simulink model "duality"  (Simulink 7.3)
settings: Solver=FixedStepDiscrete  StartTime=0.0  StopTime=10.0  FixedStep=0.02  RelTol=1e-3
libraries: voderiv x8
settings Model: Creator=Dominik  LastModifiedBy=dominik

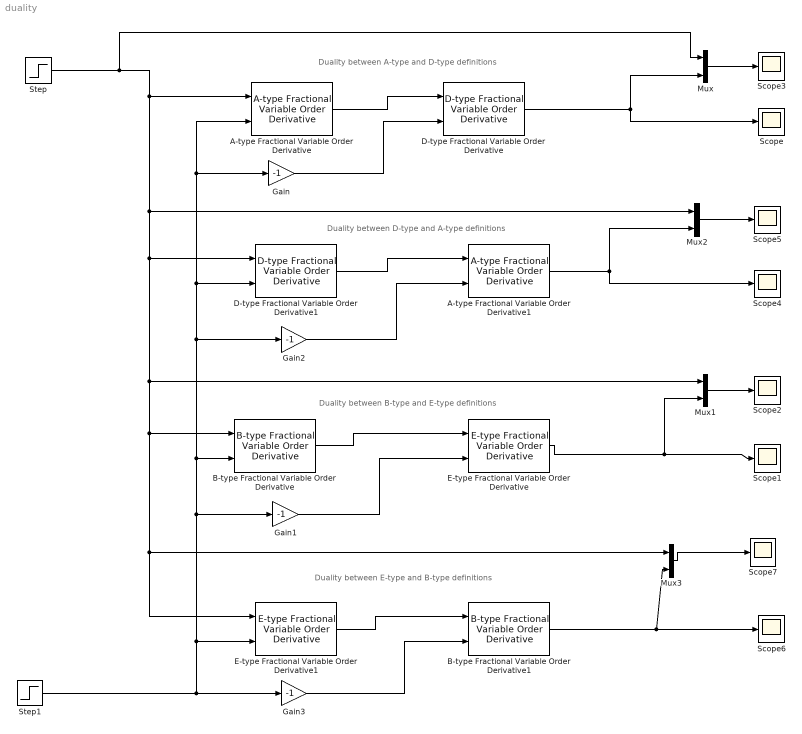
== system duality ==
  note: Duality between A-type and D-type definitions
  note: Duality between D-type and A-type definitions
  note: Duality between B-type and E-type definitions
  note: Duality between E-type and B-type definitions
  A-type Fractional Variable Order Derivative : voderiv/A-type Fractional Variable Order Derivative  N=1  Nbuf=500  Ts=0.02
  A-type Fractional Variable Order Derivative1 : voderiv/A-type Fractional Variable Order Derivative  N=1  Nbuf=500  Ts=0.02
  B-type Fractional Variable Order Derivative : voderiv/B-type Fractional Variable Order Derivative  N=1  Nbuf=500  Ts=0.02
  B-type Fractional Variable Order Derivative1 : voderiv/B-type Fractional Variable Order Derivative  N=1  Nbuf=500  Ts=0.02
  D-type Fractional Variable Order Derivative : voderiv/D-type Fractional Variable Order Derivative  N=1  Nbuf=500  Ts=0.02
  D-type Fractional Variable Order Derivative1 : voderiv/D-type Fractional Variable Order Derivative  N=1  Nbuf=500  Ts=0.02
  E-type Fractional Variable Order Derivative : voderiv/E-type Fractional Variable Order Derivative  N=1  Nbuf=500  Ts=0.02
  E-type Fractional Variable Order Derivative1 : voderiv/E-type Fractional Variable Order Derivative  N=1  Nbuf=500  Ts=0.02
  Gain{,1..3} (4 alike) : Gain  Gain=-1
  Mux{,1..3} (4 alike) : Mux  Inputs=2
  Scope{,1..7} (8 alike) : Scope
      Scope2 settings: SaveName=ScopeData2
      Scope3 settings: SaveName=ScopeData3
      Scope4 settings: SaveName=ScopeData4
      Scope5 settings: SaveName=ScopeData5
      Scope6 settings: SaveName=ScopeData6
      Scope7 settings: SaveName=ScopeData7
  Step : Step  SampleTime=0
  Step1 : Step  Time=5  Before=-0.5  After=-0.8  SampleTime=0
  wires:
  Step/1 -> Mux3/1, E-type Fractional Variable Order Derivative1/1, B-type Fractional Variable Order Derivative/1, Mux1/1, D-type Fractional Variable Order Derivative1/1, Mux2/1, A-type Fractional Variable Order Derivative/1, Mux/1
  Step1/1 -> Gain3/1, E-type Fractional Variable Order Derivative1/2, Gain1/1, Gain2/1, Gain/1, A-type Fractional Variable Order Derivative/2, D-type Fractional Variable Order Derivative1/2, B-type Fractional Variable Order Derivative/2
  Gain/1 -> D-type Fractional Variable Order Derivative/2
  Gain1/1 -> E-type Fractional Variable Order Derivative/2
  B-type Fractional Variable Order Derivative/1 -> E-type Fractional Variable Order Derivative/1
  A-type Fractional Variable Order Derivative/1 -> D-type Fractional Variable Order Derivative/1
  D-type Fractional Variable Order Derivative/1 -> Scope/1, Mux/2
  E-type Fractional Variable Order Derivative/1 -> Scope1/1, Mux1/2
  Mux1/1 -> Scope2/1
  Mux/1 -> Scope3/1
  Gain2/1 -> A-type Fractional Variable Order Derivative1/2
  D-type Fractional Variable Order Derivative1/1 -> A-type Fractional Variable Order Derivative1/1
  Mux2/1 -> Scope5/1
  A-type Fractional Variable Order Derivative1/1 -> Mux2/2, Scope4/1
  E-type Fractional Variable Order Derivative1/1 -> B-type Fractional Variable Order Derivative1/1
  Mux3/1 -> Scope7/1
  B-type Fractional Variable Order Derivative1/1 -> Mux3/2, Scope6/1
  Gain3/1 -> B-type Fractional Variable Order Derivative1/2
